simulink model "power_depletion_model"  (R2021a)
settings: Solver=FixedStepDiscrete  StartTime=0.0  StopTime=21600  FixedStep=dt  RelTol=1e-3
values from neighbouring files (symbols this model uses):
  dt = Simulink.Parameter(0.1)    [power_depletion_model.m]
settings Model: Creator=User  LastModifiedBy=User

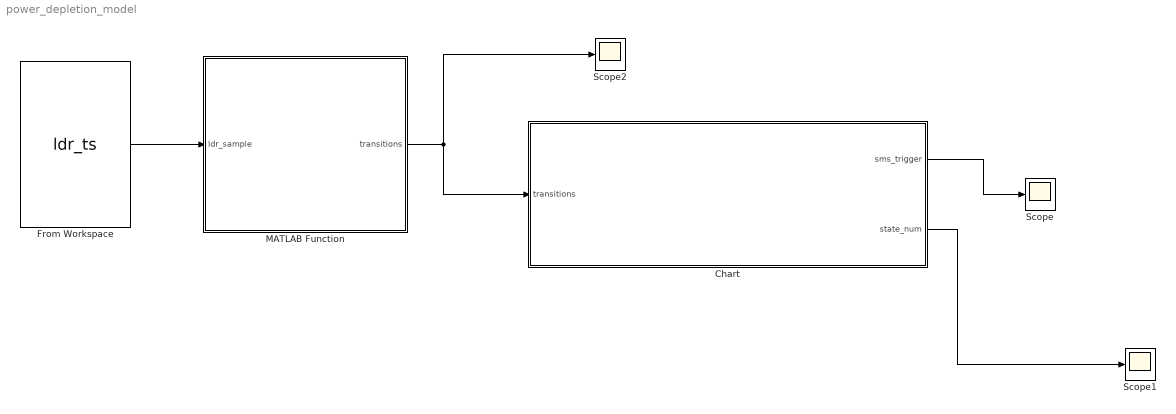
== system power_depletion_model ==
  Chart : Stateflow chart  TreatAsAtomicUnit=on
  From Workspace : FromWorkspace  VariableName=ldr_ts  SampleTime=dt
  MATLAB Function : MATLAB Function  TreatAsAtomicUnit=on
  Scope : Scope
  Scope1 : Scope
  Scope2 : Scope
  wires:
  From Workspace/1 -> MATLAB Function/1(ldr_sample)
  MATLAB Function/1(transitions) -> Chart/1(transitions), Scope2/1
  Chart/1(sms_trigger) -> Scope/1
  Chart/2(state_num) -> Scope1/1

== matlab function power_depletion_model/MATLAB Function ==
  data: ldr_sample input; transitions output

   function transitions = transitionCounter(ldr_sample)
       persistent buffer
       if isempty(buffer)
           buffer = zeros(1, 30);   % 30 = WINDOW_TICKS at dt=0.1s
       end
       buffer = [buffer(2:end), ldr_sample];
       transitions = sum(abs(diff(buffer)));
   end

== stateflow chart power_depletion_model/Chart ==
  state Monitoring
    entry: sms_trigger = 0; state_num = 1;
  state Confirmed
    entry: sms_trigger = 1; state_num = 2; cooldown_timer = 144000;
  state Cooldown
    entry: sms_trigger = 0; state_num = 3;
    during: cooldown_timer = cooldown_timer - 1;
  (default) -> Monitoring
  Monitoring -> Confirmed : [transitions >= 4]
  Confirmed -> Cooldown : after(1, tick)
  Cooldown -> Monitoring : [cooldown_timer <= 0]
  data: transitions input double; sms_trigger output double =0; cooldown_timer local double =0; state_num output double =0
